simulink model "pedestrian"  (R2024a)
settings: Solver=FixedStepAuto  StartTime=0.0  StopTime=10.0  FixedStep=0.1  RelTol=1e-3
settings Model: Creator=amir  LastModifiedBy=amir

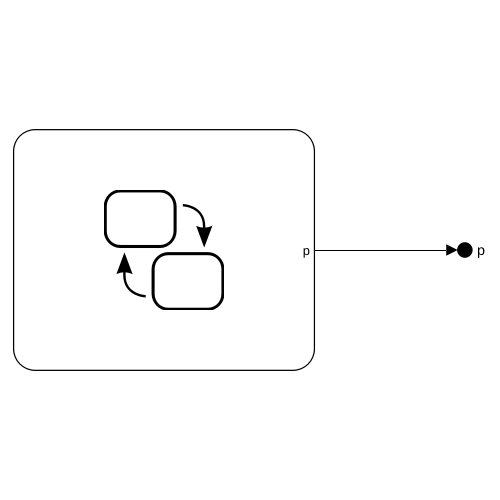
[thumbnail: Simulink's stored preview of the top-level diagram]
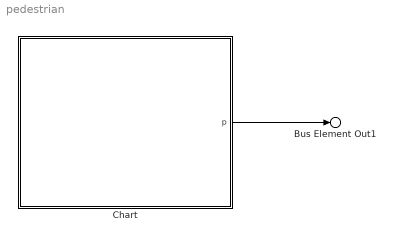
== system pedestrian ==
  Chart : Stateflow chart  TreatAsAtomicUnit=on
  Bus Element Out1 : Outport  PortName=p
  wires:
  Chart/1(p) -> Bus Element Out1/1

== stateflow chart pedestrian/Chart ==
  state Idle
    p=0
  state WantsToPass
    p=1
  (default) -> Idle : {cnt=0}
  WantsToPass -> WantsToPass [order 2] : {cnt = cnt+1}
  Idle -> Idle [order 2] : {cnt = cnt+1}
  Idle -> WantsToPass [order 1] : [cnt == 60]{cnt = 0}
  WantsToPass -> Idle [order 1] : [cnt == 120]{cnt = 0}
  data: p output; cnt local
